simulink model "cascade"  (R2015a)
settings: Solver=ode45  StartTime=0.0  StopTime=10  RelTol=1e-3
libraries: powerlib x23, powerlib_meascontrol x1
settings Model: Creator=Kelvin Gakuo  LastModifiedBy=Kelvin Gakuo

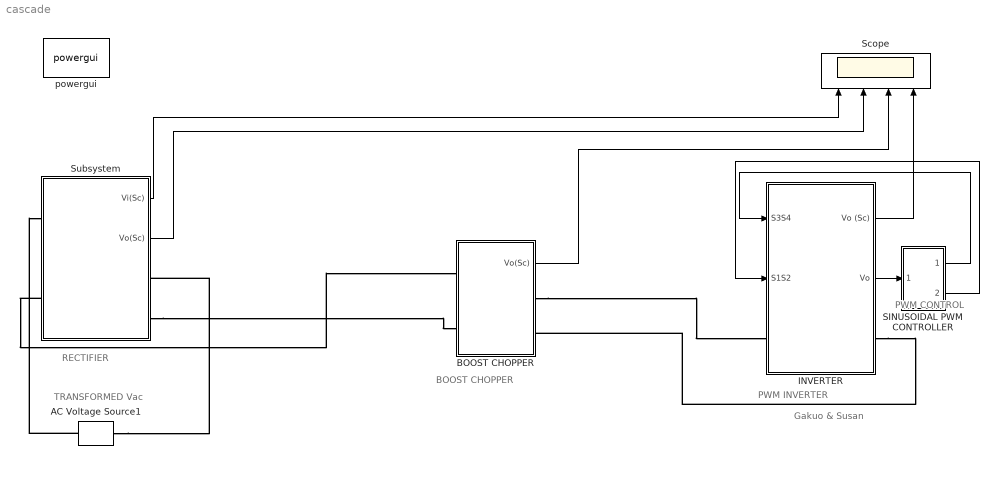
== system cascade ==
  note: TRANSFORMED Vac
  note: RECTIFIER
  note: Gakuo & Susan
  note: PWM CONTROL
  note: PWM INVERTER
  note: BOOST CHOPPER
  AC Voltage Source1 : powerlib/Electrical Sources/AC Voltage Source  Amplitude=40.84  Phase=0  Frequency=50  SampleTime=0  Measurements=None
  BOOST CHOPPER : Subsystem
  INVERTER : Subsystem
  SINUSOIDAL PWM CONTROLLER : Subsystem
  Scope : Scope  NumInputPorts=4
      settings: TimeRange=0.1  YMin=-50~-5~0~-75  YMax=50~45~80~75
  Subsystem : Subsystem
  powergui : powerlib/powergui  Priority=1  SimulationMode=Continuous  SolverType=Tustin/Backward Euler (TBE)  SampleTime=50e-6  frequency=60  SPID=on  DisableSnubberDevices=off  DisableRonSwitches=off  DisableVfSwitches=off  SwTol=0  DisplayEquations=off  Interpol=off  methode=off  Ts=100  FunctionMessages=off  echomessages=off  HookPort=off  EnableUseOfTLC=off  x0status=blocks  frequencyindice=0  Pbase=100e6  ErrMax=1e-4  Iterations=50  UnitsV=kV  UnitsW=MW  buscounter=0  RestoreLinks=warning  ResistiveCurrentMeasurement=off  Frange=[0:2:500]  Ylog=off  Xlog=on  ShowGrid=off  save=off  variable=ZData  structure=0  ZoomFFT=off  StartTime=0.0  cycles=1  DisplayStyle=1  fundamental=60  FreqAxis=off  MaxFrequency=1000  frequencyindicesteady=1  RmsSteady=1  display=off
  wires:
  INVERTER/2(Vo) -> SINUSOIDAL PWM CONTROLLER/1(In1)
  SINUSOIDAL PWM CONTROLLER/1(S3S4) -> INVERTER/1(S3S4)
  SINUSOIDAL PWM CONTROLLER/2(S1S2) -> INVERTER/2(S1S2)
  Subsystem/1(Vi(Sc)) -> Scope/1
  Subsystem/2(Vo(Sc)) -> Scope/2
  BOOST CHOPPER/1(Vo(Sc)) -> Scope/3
  INVERTER/1(Vo (Sc)) -> Scope/4
  connections:
  BOOST CHOPPER/RConn1 -- INVERTER/LConn1
  INVERTER/RConn1 -- BOOST CHOPPER/RConn2
  AC Voltage Source1/LConn1 -- Subsystem/RConn1
  AC Voltage Source1/RConn1 -- Subsystem/LConn1
  Subsystem/RConn2 -- BOOST CHOPPER/LConn2
  Subsystem/LConn2 -- BOOST CHOPPER/LConn1

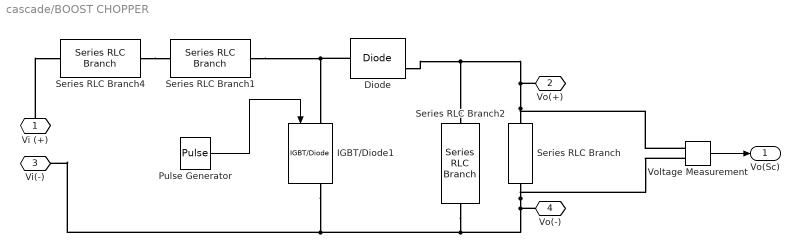
== system cascade/BOOST CHOPPER ==
  Diode : powerlib/Power Electronics/Diode  Ron=0.001  Lon=0  Vf=0.8  IC=0  UseSnubber=off  Rs=500  Cs=250e-9  Measurements=on
  IGBT/Diode1 : powerlib/Power Electronics/IGBT//Diode  Ron=1e-3  Rs=1e5  Cs=inf  Measurements=on
  Pulse Generator : DiscretePulseGenerator  PulseType=Time based  Amplitude=10  Period=2e-5  PulseWidth=40
  Series RLC Branch : powerlib/Elements/Series RLC Branch  LConnTagsString=__new0  RConnTagsString=__new0  BranchType=R  Resistance=47.5  Inductance=1e-3  SetiL0=off  InitialCurrent=0  Capacitance=1e-6  Setx0=off  InitialVoltage=0  Measurements=None
  Series RLC Branch1 : powerlib/Elements/Series RLC Branch  LConnTagsString=__new0  RConnTagsString=__new0  BranchType=L  Resistance=100  Inductance=12e-6  SetiL0=off  InitialCurrent=0  Capacitance=0.7e-3  Setx0=off  InitialVoltage=0  Measurements=None
  Series RLC Branch2 : powerlib/Elements/Series RLC Branch  LConnTagsString=__new0  RConnTagsString=__new0  BranchType=C  Resistance=100  Inductance=120e-3  SetiL0=off  InitialCurrent=0  Capacitance=82e-6  Setx0=off  InitialVoltage=0  Measurements=None
  Series RLC Branch4 : powerlib/Elements/Series RLC Branch  LConnTagsString=__new0  RConnTagsString=__new0  BranchType=R  Resistance=0.1  Inductance=120e-3  SetiL0=off  InitialCurrent=0  Capacitance=0.7e-3  Setx0=off  InitialVoltage=0  Measurements=None
  Voltage Measurement : powerlib/Measurements/Voltage Measurement  PhasorSimulation=off  OutputType=Complex  PSBequivalent=0
  Vi (+) : PMIOPort  Port=1  Side=Left
  Vo(+) : PMIOPort  Port=2  Side=Right
  "Vi(-) " : PMIOPort  Port=3  Side=Left
  Vo(-) : PMIOPort  Port=4  Side=Right
  Vo(Sc) : Outport
  wires:
  Pulse Generator/1 -> IGBT/Diode1/1
  Voltage Measurement/1 -> Vo(Sc)/1
  connections:
  Diode/LConn1 -- Series RLC Branch1/RConn1 -- IGBT/Diode1/LConn1
  Vi (+)/RConn1 -- Series RLC Branch4/LConn1
  Series RLC Branch4/RConn1 -- Series RLC Branch1/LConn1
  Vo(+)/RConn1 -- Diode/RConn1 -- Series RLC Branch2/LConn1 -- Series RLC Branch/LConn1 -- Voltage Measurement/LConn1
  Series RLC Branch2/RConn1 -- IGBT/Diode1/RConn1 -- "Vi(-) "/RConn1 -- Series RLC Branch/RConn1 -- Voltage Measurement/LConn2 -- Vo(-)/RConn1

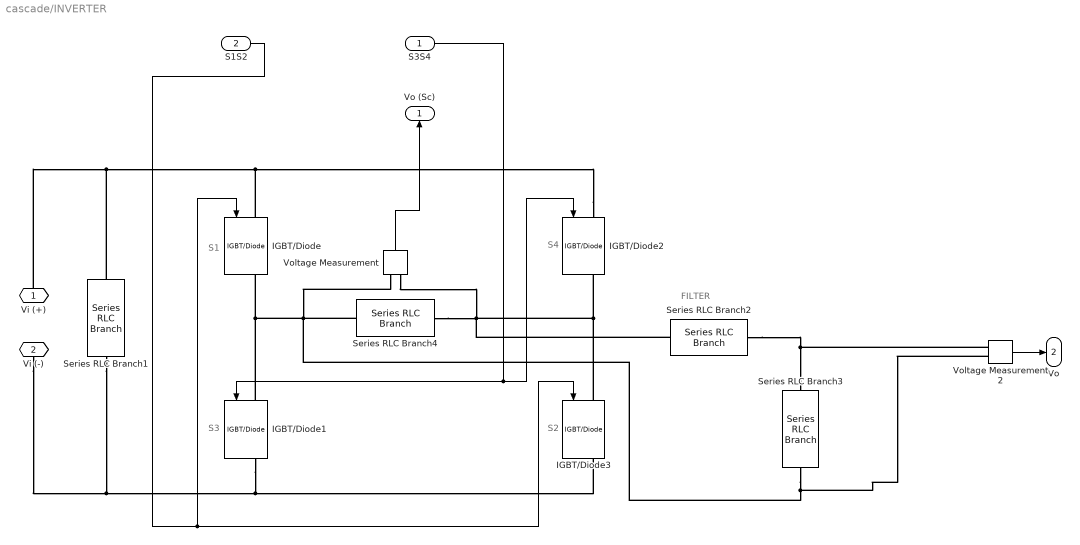
== system cascade/INVERTER ==
  note: S3
  note: S4
  note: S2
  note: S1
  note: FILTER
  S3S4 : Inport
  S1S2 : Inport  Port=2
  IGBT/Diode{,1..3} (4 alike) : powerlib/Power Electronics/IGBT//Diode  Ron=1e-3  Rs=1e5  Cs=inf  Measurements=on
  Series RLC Branch1 : powerlib/Elements/Series RLC Branch  LConnTagsString=__new0  RConnTagsString=__new0  BranchType=RC  Resistance=1  Inductance=1e-3  SetiL0=off  InitialCurrent=0  Capacitance=0.7e-3  Setx0=off  InitialVoltage=0  Measurements=None
  Series RLC Branch2 : powerlib/Elements/Series RLC Branch  LConnTagsString=__new0  RConnTagsString=__new0  BranchType=RL  Resistance=100  Inductance=120e-3  SetiL0=off  InitialCurrent=0  Capacitance=0.7e-3  Setx0=off  InitialVoltage=0  Measurements=None
  Series RLC Branch3 : powerlib/Elements/Series RLC Branch  LConnTagsString=__new0  RConnTagsString=__new0  BranchType=C  Resistance=100  Inductance=120e-3  SetiL0=off  InitialCurrent=0  Capacitance=0.7e-3  Setx0=off  InitialVoltage=0  Measurements=None
  Series RLC Branch4 : powerlib/Elements/Series RLC Branch  LConnTagsString=__new0  RConnTagsString=__new0  BranchType=R  Resistance=100  Inductance=120e-3  SetiL0=off  InitialCurrent=0  Capacitance=0.7e-3  Setx0=off  InitialVoltage=0  Measurements=None
  Voltage Measurement : powerlib/Measurements/Voltage Measurement  PhasorSimulation=off  OutputType=Complex  PSBequivalent=0
  Voltage Measurement2 : powerlib/Measurements/Voltage Measurement  PhasorSimulation=off  OutputType=Complex  PSBequivalent=0
  Vi (+) : PMIOPort  Port=1  Side=Left
  Vi (-) : PMIOPort  Port=2  Side=Right
  Vo (Sc) : Outport
  Vo : Outport  Port=2
  wires:
  Voltage Measurement/1 -> Vo (Sc)/1
  S3S4/1 -> IGBT/Diode2/1, IGBT/Diode1/1
  S1S2/1 -> IGBT/Diode3/1, IGBT/Diode/1
  Voltage Measurement2/1 -> Vo/1
  connections:
  IGBT/Diode3/RConn1 -- IGBT/Diode1/RConn1 -- Vi (-)/RConn1 -- Series RLC Branch1/LConn1
  IGBT/Diode2/RConn1 -- IGBT/Diode3/LConn1 -- Series RLC Branch2/RConn1 -- Voltage Measurement/LConn2 -- Series RLC Branch4/RConn1
  IGBT/Diode1/LConn1 -- IGBT/Diode/RConn1 -- Voltage Measurement2/LConn2 -- Series RLC Branch3/RConn1 -- Series RLC Branch4/LConn1 -- Voltage Measurement/LConn1
  Series RLC Branch2/LConn1 -- Series RLC Branch3/LConn1 -- Voltage Measurement2/LConn1
  IGBT/Diode2/LConn1 -- IGBT/Diode/LConn1 -- Vi (+)/RConn1 -- Series RLC Branch1/RConn1

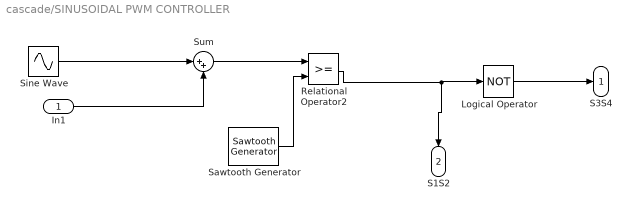
== system cascade/SINUSOIDAL PWM CONTROLLER ==
  In1 : Inport
  Logical Operator : Logic  Operator=NOT  AllPortsSameDT=off  OutDataTypeStr=boolean
  Relational Operator2 : RelationalOperator  OutDataTypeStr=boolean  ZeroCross=off
  Sawtooth Generator : powerlib_meascontrol/Pulse & Signal Generators/Sawtooth Generator  Freq=80  Phase=180  Ts=0
  Sine Wave : Sin  Frequency=2*pi*80  SampleTime=0
  Sum : Sum  Inputs=|++
  S3S4 : Outport
  S1S2 : Outport  Port=2
  wires:
  In1/1 -> Sum/2
  Sawtooth Generator/1 -> Relational Operator2/2
  Sum/1 -> Relational Operator2/1
  Logical Operator/1 -> S3S4/1
  Sine Wave/1 -> Sum/1
  Relational Operator2/1 -> S1S2/1, Logical Operator/1

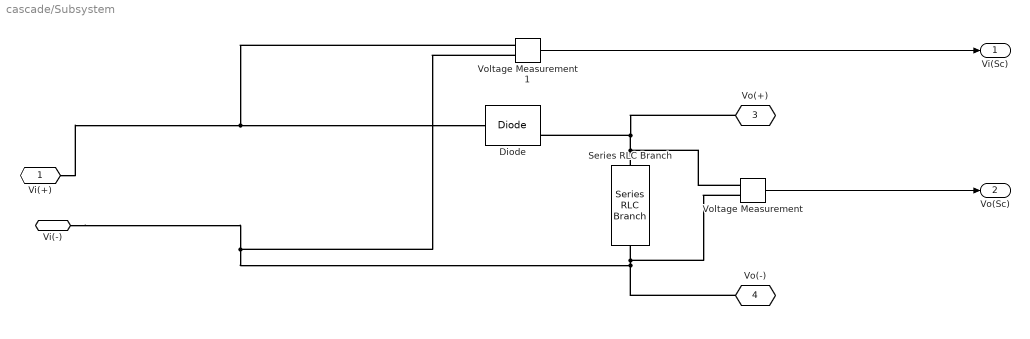
== system cascade/Subsystem ==
  Diode : powerlib/Power Electronics/Diode  Ron=0.001  Lon=0  Vf=0.8  IC=0  UseSnubber=off  Rs=500  Cs=250e-9  Measurements=on
  Series RLC Branch : powerlib/Elements/Series RLC Branch  LConnTagsString=__new0  RConnTagsString=__new0  BranchType=R  Resistance=40.81  Inductance=1e-3  SetiL0=off  InitialCurrent=0  Capacitance=1e-6  Setx0=off  InitialVoltage=0  Measurements=None
  Voltage Measurement : powerlib/Measurements/Voltage Measurement  PhasorSimulation=off  OutputType=Complex  PSBequivalent=0
  Voltage Measurement1 : powerlib/Measurements/Voltage Measurement  PhasorSimulation=off  OutputType=Complex  PSBequivalent=0
  Vi(+) : PMIOPort  Port=1  Side=Left
  Vi(-) : PMIOPort  Port=2  Side=Right
  Vo(+) : PMIOPort  Port=3  Side=Left
  Vo(-) : PMIOPort  Port=4  Side=Right
  Vi(Sc) : Outport
  Vo(Sc) : Outport  Port=2
  wires:
  Voltage Measurement/1 -> Vo(Sc)/1
  Voltage Measurement1/1 -> Vi(Sc)/1
  connections:
  Voltage Measurement1/LConn1 -- Diode/LConn1 -- Vi(+)/RConn1
  Voltage Measurement1/LConn2 -- Voltage Measurement/LConn2 -- Series RLC Branch/RConn1 -- Vo(-)/RConn1 -- Vi(-)/RConn1
  Series RLC Branch/LConn1 -- Vo(+)/RConn1 -- Diode/RConn1 -- Voltage Measurement/LConn1
